simulink model "simulacao"  (Simulink 8.5)
settings: Solver=ode4  SolverMode=SingleTasking  StartTime=0.0  StopTime=80  FixedStep=0.001  RelTol=1e-3
InitFcn:
  | alpha = 20.70;
  | beta =  1.27;
  | gamma = 0.53;
values from neighbouring files (symbols this model uses):
  Kd_pid1 = gains(3)    [projeto.m]
  Kd_pid2 = gains(3)    [projeto.m]
  Kd_pid3 = gains(3)    [projeto.m]
  Kd_pid4 = gains(3)    [projeto.m]
  Kd_pid5 = gains(3)    [projeto.m]
  Ki_pid1 = gains(2)    [projeto.m]
  Ki_pid2 = gains(2)    [projeto.m]
  Ki_pid3 = gains(2)    [projeto.m]
  Ki_pid4 = gains(2)    [projeto.m]
  Ki_pid5 = gains(2)    [projeto.m]
  Kp_pid1 = gains(1)    [projeto.m]
  Kp_pid2 = gains(1)    [projeto.m]
  Kp_pid3 = gains(1)    [projeto.m]
  Kp_pid4 = gains(1)    [projeto.m]
  Kp_pid5 = gains(1)    [projeto.m]
  N_pid1 = 20    [projeto.m]
  N_pid2 = 20    [projeto.m]
  N_pid3 = 21    [projeto.m]
  N_pid4 = 21    [projeto.m]
  N_pid5 = 21    [projeto.m]
undefined symbols (not defined in the file or in its folder): sigbuilder_block
libraries: simulink_extras x2, simulink x1
settings Model: Creator=colom  LastModifiedBy=colom  SimulationMode=accelerator  CovMetricSettings=dwe  CovHtmlReporting=off  covSaveCumulativeToWorkspaceVar=off  CovSaveSingleToWorkspaceVar=off  CovExternalEMLEnable=on
settings SolverCC: AutoInsertRateTranBlk=on
settings DataIOCC: LimitDataPoints=off  SaveFormat=Dataset  SignalLoggingSaveFormat=Dataset  ReturnWorkspaceOutputs=on
settings OptimizationCC: ExpressionDepthLimit=128
settings DebuggingCC: UnderspecifiedInitializationDetection=Simplified  MergeDetectMultiDrivingBlocksExec=error  FcnCallInpInsideContextMsg=EnableAllAsError  UnconnectedInputMsg=none  UnconnectedOutputMsg=none  UnconnectedLineMsg=none  StateNameClashWarn=none  SFUnexpectedBacktrackingDiag=error  SFNoUnconditionalDefaultTransitionDiag=error
settings HardwareCC: ProdBitPerPointer=64  ProdLargestAtomicFloat=Float  ProdIntDivRoundTo=Zero  ProdEndianess=LittleEndian  ProdHWDeviceType=Specified
settings ModelReferenceCC: PropagateSignalLabelsOutOfModel=on
settings SFSimCC: SimUseLocalCustomCode=on
settings RTWCC: RTWUseLocalCustomCode=on
settings GRTTargetCC: TargetLangStandard=C99 (ISO)  CombineOutputUpdateFcns=on  GRTInterface=off

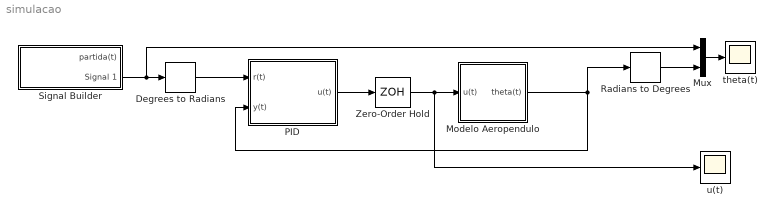
== system simulacao ==
  Degrees to Radians : simulink_extras/Transformations/Degrees to Radians
  Modelo Aeropendulo : Subsystem
  Mux : Mux  Inputs=2
  PID : Subsystem
  Radians to Degrees : simulink_extras/Transformations/Radians to Degrees
  Signal Builder : Subsystem  Tag=STV Subsys  LoadFcn=sigbuilder_block('load',[302.25 165 1093.5 399.75 ]);  StartFcn=sigbuilder_block('start');  StopFcn=sigbuilder_block('stop');  ClipboardFcn=sigbuilder_block('clipboard');  mask(Sigbuilder block){}
      mask help: Simulink:masks:SigbuilderBlock_MD
      mask init:
      | if ~strcmp(get_param(bdroot(gcbh),'SimulationStatus'),'stopped') tuvar = sigbuilder_block('maskInit'); end
      settings: CopyFcn=sigbuilder_block('copy');  DeleteFcn=sigbuilder_block('delete');  ModelCloseFcn=sigbuilder_block('modelClose');  PreSaveFcn=sigbuilder_block('preSave');  PauseFcn=sigbuilder_block('pause');  ContinueFcn=sigbuilder_block('continue');  NameChangeFcn=sigbuilder_block('namechange');  OpenFcn=sigbuilder_block('open',[302.25 165 1093.5 399.75 ]);  CloseFcn=sigbuilder_block('close');
      mask Display: plot(0, 0, 100, 100,[2, 2, 32, 32, 2], [68, 8, 8, 68, 68],[32, 2], [38, 38], [32, 19, 2],[53, 60, 44], [32, 17, 17, 2],[16, 16, 31, 31]);txt = getActiveGroup(gcbh);text(2, 100, txt,'verticalAlignment', 'top');
  Zero-Order Hold : ZeroOrderHold  SampleTime=0.010
  theta(t) : Scope
      settings: TimeRange=80  YMin=-0.0001795191898532442  YMax=100
  u(t) : Scope
      settings: TimeRange=40  YMin=-10  YMax=20
  wires:
  Zero-Order Hold/1 -> Modelo Aeropendulo/1(u(t)), u(t)/1
  PID/1(u(t)) -> Zero-Order Hold/1
  Modelo Aeropendulo/1(theta(t)) -> Radians to Degrees/1, PID/2(y(t))
  Degrees to Radians/1 -> PID/1(r(t))
  Signal Builder/2(Signal 1) -> Mux/1, Degrees to Radians/1
  Mux/1 -> theta(t)/1
  Radians to Degrees/1 -> Mux/2

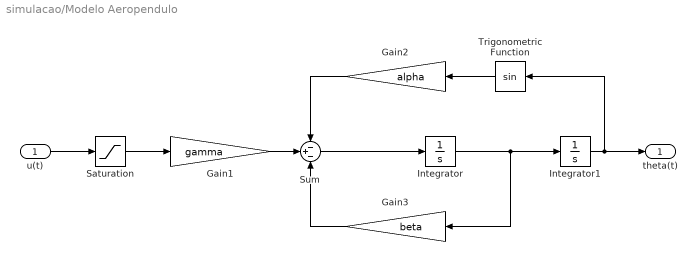
== system simulacao/Modelo Aeropendulo ==
  u(t) : Inport
  Gain1 : Gain  Gain=gamma
  Gain2 : Gain  Gain=alpha
  Gain3 : Gain  Gain=beta
  Integrator : Integrator
  Integrator1 : Integrator
  Saturation : Saturate  UpperLimit=100  LowerLimit=0
  Sum : Sum  Inputs=-+-
  Trigonometric Function : Trigonometry
  theta(t) : Outport
  wires:
  Gain3/1 -> Sum/3
  u(t)/1 -> Saturation/1
  Integrator1/1 -> theta(t)/1, Trigonometric Function/1
  Trigonometric Function/1 -> Gain2/1
  Gain2/1 -> Sum/1
  Integrator/1 -> Gain3/1, Integrator1/1
  Sum/1 -> Integrator/1
  Gain1/1 -> Sum/2
  Saturation/1 -> Gain1/1

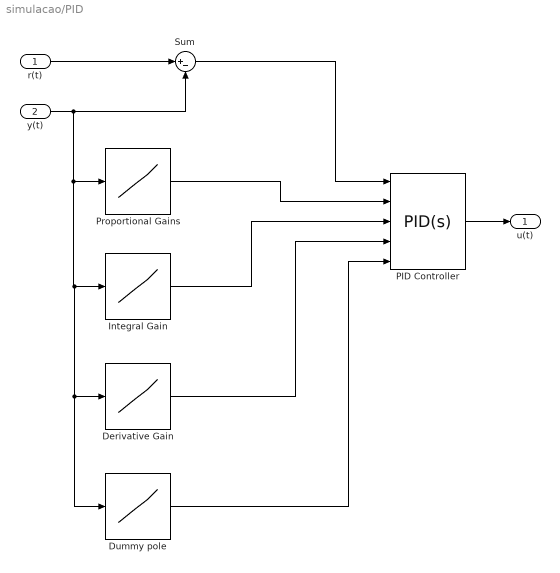
== system simulacao/PID ==
  r(t) : Inport
  y(t) : Inport  Port=2
  Derivative Gain : Lookup_n-D  NumberOfTableDimensions=1  BreakpointsForDimension1=deg2rad([15 37.5 55 70 85])  BreakpointsForDimension2=[-5:5]  BreakpointsForDimension3=[-5:5]  BreakpointsForDimension4=[-5:5]  Table=[Kd_pid1 Kd_pid2 Kd_pid3 Kd_pid4 Kd_pid5]  InternalRulePriority=Speed  RndMeth=Simplest  InputSameDT=on
  Dummy pole : Lookup_n-D  NumberOfTableDimensions=1  BreakpointsForDimension1=deg2rad([15 37.5 55 70 85])  BreakpointsForDimension2=[-5:5]  BreakpointsForDimension3=[-5:5]  BreakpointsForDimension4=[-5:5]  Table=[N_pid1 N_pid2 N_pid3 N_pid4 N_pid5]  InternalRulePriority=Speed  RndMeth=Simplest  InputSameDT=on
  Integral Gain : Lookup_n-D  NumberOfTableDimensions=1  BreakpointsForDimension1=deg2rad([15 37.5 55 70 85])  BreakpointsForDimension2=[-5:5]  BreakpointsForDimension3=[-5:5]  BreakpointsForDimension4=[-5:5]  Table=[Ki_pid1 Ki_pid2 Ki_pid3 Ki_pid4 Ki_pid5]  InternalRulePriority=Speed  RndMeth=Simplest  InputSameDT=on
  PID Controller : simulink/Continuous/PID Controller  Controller=PID  TimeDomain=Continuous-time  SampleTime=-1  IntegratorMethod=Forward Euler  FilterMethod=Forward Euler  Form=Parallel  UseFilter=on  ControllerParametersSource=external  P=1  I=1  D=0  N=100  InitialConditionSource=internal  InitialConditionForIntegrator=0  InitialConditionForFilter=0  ExternalReset=none  LimitOutput=off  UpperSaturationLimit=inf  LowerSaturationLimit=-inf  LinearizeAsGain=on  AntiWindupMode=none  Kb=1  TrackingMode=off  Kt=1  PParamMin=[]  PParamMax=[]  IParamMin=[]  IParamMax=[]  DParamMin=[]  DParamMax=[]  NParamMin=[]  NParamMax=[]  KbParamMin=[]  KbParamMax=[]  KtParamMin=[]  KtParamMax=[]  POutMin=[]  POutMax=[]  IOutMin=[]  IOutMax=[]  DOutMin=[]  DOutMax=[]  NOutMin=[]  NOutMax=[]  KbOutMin=[]  KbOutMax=[]  KtOutMin=[]  KtOutMax=[]  IntegratorOutMin=[]  IntegratorOutMax=[]  FilterOutMin=[]  FilterOutMax=[]  SumOutMin=[]  SumOutMax=[]  SumI1OutMin=[]  SumI1OutMax=[]  SumI2OutMin=[]  SumI2OutMax=[]  SumI3OutMin=[]  SumI3OutMax=[]  SumDOutMin=[]  SumDOutMax=[]  SaturationOutMin=[]  SaturationOutMax=[]  IntegratorContinuousStateAttributes=''  IntegratorStateMustResolveToSignalObject=off  IntegratorRTWStateStorageClass=Auto  FilterContinuousStateAttributes=''  FilterStateMustResolveToSignalObject=off  FilterRTWStateStorageClass=Auto  DifferentiatorICPrevScaledInput=0  DifferentiatorOutMin=[]  DifferentiatorOutMax=[]
  Proportional Gains : Lookup_n-D  NumberOfTableDimensions=1  BreakpointsForDimension1=deg2rad([15 37.5 55 70 85])  BreakpointsForDimension2=[-5:5]  BreakpointsForDimension3=[-5:5]  BreakpointsForDimension4=[-5:5]  Table=[Kp_pid1 Kp_pid2 Kp_pid3 Kp_pid4 Kp_pid5]  InternalRulePriority=Speed  RndMeth=Simplest  InputSameDT=on
  Sum : Sum  Inputs=|+-
  u(t) : Outport
  wires:
  y(t)/1 -> Dummy pole/1, Derivative Gain/1, Integral Gain/1, Proportional Gains/1, Sum/2
  r(t)/1 -> Sum/1
  PID Controller/1 -> u(t)/1
  Dummy pole/1 -> PID Controller/5
  Proportional Gains/1 -> PID Controller/2
  Sum/1 -> PID Controller/1
  Integral Gain/1 -> PID Controller/3
  Derivative Gain/1 -> PID Controller/4

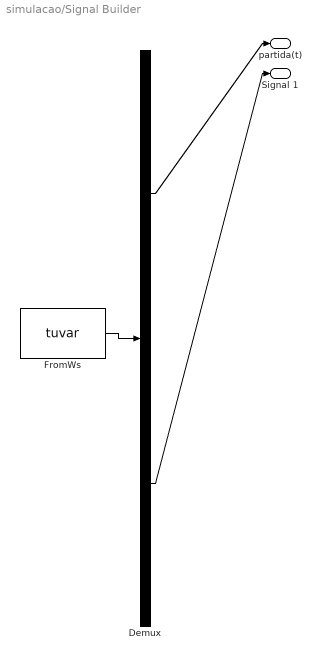
== system simulacao/Signal Builder ==
  Demux : Demux  Tag=STV Demux  Outputs=2
  FromWs : FromWorkspace  Tag=STV FromWs  VariableName=tuvar  SampleTime=0  SigBuilderData=DataTag0  VnvData=DataTag1
      SigBuilderData=|
      | common.afterFinalStr = 'Extrapolate'
      | common.sampleTime = 0
      | dataSet.timeRange = [0 80]
      | dataSet.name = 'Group 1'
      | sbobj.Groups.Name = 'Group 1'
      | sbobj.Groups.Signals(1).Name = 'partida(t)'
      | sbobj.Groups.Signals(1).XData = [0 0.5 0.5 2.5 2.5 6.5 6.5 10 10 15 16 17 18 19 80]
      | sbobj.Groups.Signals(1).YData = [0 0 2000 2000 2 0 1040 1040 4 0 0 0 0 0 0]
      | sbobj.Groups.Signals(2).Name = 'Signal 1'
      | sbobj.Groups.Signals(2).XData = [0 11 15 20 23 28 31 36 39 44 44 47 52 52 72 73 74 75 76 77 78 79 80]
      | sbobj.Groups.Signals(2).YData = [0 0 20 20 40 40 60 60 75 75 85 85 85 75 0 0 0 0 0 0 0 0 0]
      | sbobj.Groups.TimeRange = [0 80]
  partida(t) : Outport  Tag=STV Outport
  Signal 1 : Outport  Tag=STV Outport  Port=2
  wires:
  FromWs/1 -> Demux/1
  Demux/1 -> partida(t)/1
  Demux/2 -> Signal 1/1
